simulink model "test_delay"  (R2023b)
settings: Solver=FixedStepAuto  StartTime=0.0  StopTime=30  FixedStep=0.001  RelTol=1e-3
libraries: sensors_subsystems x1
settings Model: Creator=brent  LastModifiedBy=brent

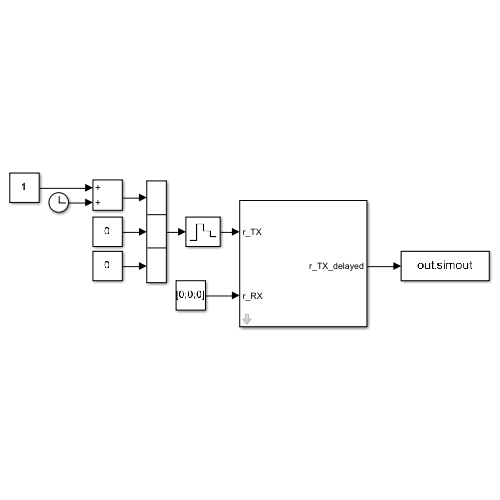
[thumbnail: Simulink's stored preview of the top-level diagram]
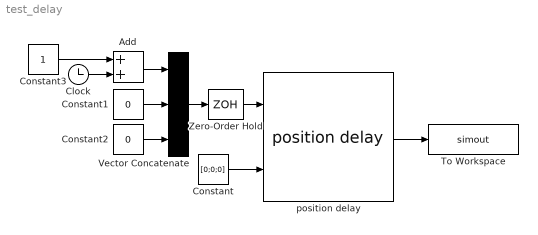
== system test_delay ==
  Add : Sum
  Clock : Clock
  Constant : Constant  Value=[0;0;0]
  Constant1 : Constant  Value=0
  Constant2 : Constant  Value=0
  Constant3 : Constant
  To Workspace : ToWorkspace  VariableName=simout  SaveFormat=Timeseries  SampleTime=-1
  Vector Concatenate : Concatenate  NumInputs=3
  Zero-Order Hold : ZeroOrderHold  SampleTime=10
  position delay : sensors_subsystems/position delay  light_speed=10  sample_time=10
      settings: SourceProductName=Sensors library
  wires:
  Constant/1 -> position delay/2
  position delay/1 -> To Workspace/1
  Constant1/1 -> Vector Concatenate/2
  Constant2/1 -> Vector Concatenate/3
  Clock/1 -> Add/2
  Constant3/1 -> Add/1
  Add/1 -> Vector Concatenate/1
  Vector Concatenate/1 -> Zero-Order Hold/1
  Zero-Order Hold/1 -> position delay/1
